simulink model "adcs_sensors"  (R2024b)
settings: Solver=VariableStepAuto  StartTime=0.0  StopTime=10.0  RelTol=1e-3
undefined symbols (not defined in the file): gyro_arw, gyro_bias_instab, sun_dir_inertial
libraries: simulink x2
settings Model: DataDictionary=adcs_params.sldd  Creator=natha  LastModifiedBy=natha

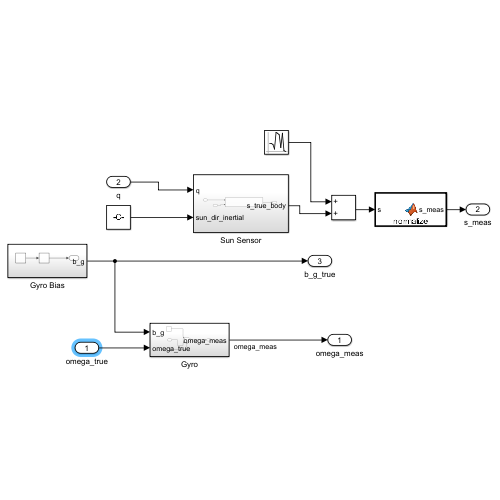
[thumbnail: Simulink's stored preview of the top-level diagram]
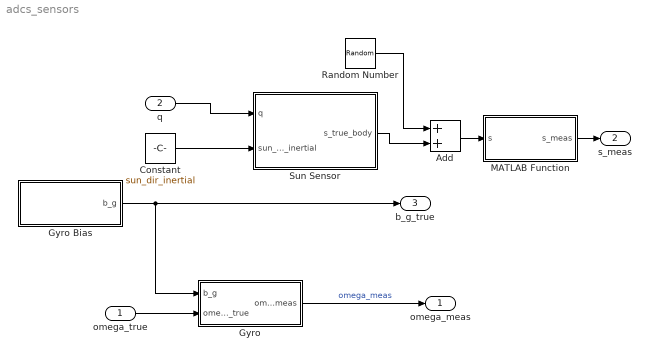
== system adcs_sensors ==
  omega_true : Inport  PortDimensions=[3 1]
  q : Inport  Port=2
  Add : Sum
  Constant : Constant  Value=sun_dir_inertial
  Gyro : Subsystem
  Gyro Bias : Subsystem
  MATLAB Function : MATLAB Function  TreatAsAtomicUnit=on
  Random Number : RandomNumber  Variance=(0.5*pi/180)^2  SampleTime=0.01
  Sun Sensor : Subsystem
  omega_meas : Outport
  s_meas : Outport  Port=2
  b_g_true : Outport  Port=3
  wires:
  Gyro/1(omega_meas) -> omega_meas/1  "omega_meas"
  Gyro Bias/1(b_g) -> b_g_true/1, Gyro/1(b_g)
  Constant/1 -> Sun Sensor/2(sun_dir_inertial)
  omega_true/1 -> Gyro/2(omega_true)
  q/1 -> Sun Sensor/1(q)
  Random Number/1 -> Add/1
  Sun Sensor/1(s_true_body) -> Add/2
  Add/1 -> MATLAB Function/1(s)
  MATLAB Function/1(s_meas) -> s_meas/1

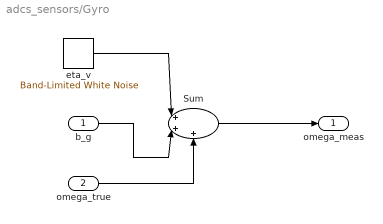
== system adcs_sensors/Gyro ==
  b_g : Inport
  omega_true : Inport  Port=2
  Sum : Sum  Inputs=|+++
  eta_v : simulink/Sources/Band-Limited White Noise  Cov=gyro_arw^2  Ts=0.01  seed=[23341]
  omega_meas : Outport
  wires:
  eta_v/1 -> Sum/1
  b_g/1 -> Sum/2
  omega_true/1 -> Sum/3
  Sum/1 -> omega_meas/1

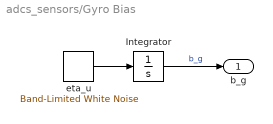
== system adcs_sensors/Gyro Bias ==
  Integrator : Integrator  InitialCondition=2.4e-6
  eta_u : simulink/Sources/Band-Limited White Noise  Cov=(gyro_bias_instab/60)^2  Ts=0.1  seed=[23341]
  b_g : Outport
  wires:
  eta_u/1 -> Integrator/1
  Integrator/1 -> b_g/1  "b_g"

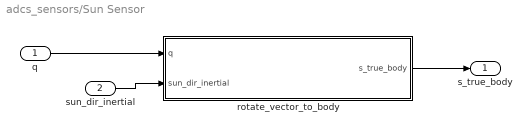
== system adcs_sensors/Sun Sensor ==
  q : Inport  PortDimensions=[4 1]
  sun_dir_inertial : Inport  Port=2
  rotate_vector_to_body : MATLAB Function  TreatAsAtomicUnit=on
  s_true_body : Outport
  wires:
  q/1 -> rotate_vector_to_body/1(q)
  sun_dir_inertial/1 -> rotate_vector_to_body/2(sun_dir_inertial)
  rotate_vector_to_body/1(s_true_body) -> s_true_body/1

== matlab function adcs_sensors/Sun Sensor/rotate_vector_to_body ==
  data: q input; s_true_body output; sun_dir_inertial input
function s_true_body = rotate_vector_to_body(q,sun_dir_inertial)

DCM = [1-2*(q(2)^2+q(3)^2) 2*(q(1)*q(2)+q(3)*q(4)) 2*(q(1)*q(3)-q(2)*q(4));
       2*(q(1)*q(2)-q(3)*q(4)) 1-2*(q(1)^2+q(3)^2) 2*(q(2)*q(3)+q(1)*q(4));
       2*(q(1)*q(3)+q(2)*q(4)) 2*(q(2)*q(3)-q(1)*q(4)) 1-2*(q(1)^2+q(2)^2)];

s_true_body = DCM * sun_dir_inertial;

== matlab function adcs_sensors/MATLAB Function ==
  data: s input; s_meas output
function s_meas = normalize(s)

s_meas = s / norm(s);
